simulink model "L_vs_pos_host"  (R2021b)
settings: Solver=ode1  StartTime=0.0  StopTime=inf  FixedStep=1e-3  RelTol=1e-3
InitFcn:
  | X_to_L = 1/(20*2*pi);
libraries: slrealtimeutilitieslib x1, slrealtimeiplib x1, simulink x1
settings Model: Creator=tcraddoc  LastModifiedBy=wasynczu
settings SolverCC: AlgebraicLoopSolver=TrustRegion
settings DataIOCC: ReturnWorkspaceOutputs=off
settings DebuggingCC: SFMachineParentedDataDiag=warning  ArithmeticOperatorsInVariantConditions=warning
settings SFSimCC: SimUseLocalCustomCode=off  CustomCodeUndefinedFunction=UseInterfaceOnly
settings RTWCC: RTWUseLocalCustomCode=off
settings CodeAppCC: StateflowObjectComments=on

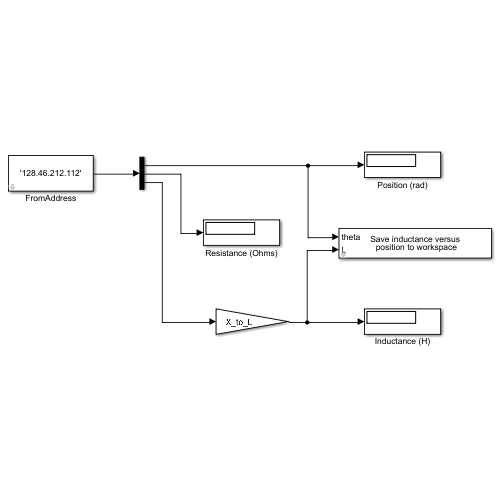
[thumbnail: Simulink's stored preview of the top-level diagram]
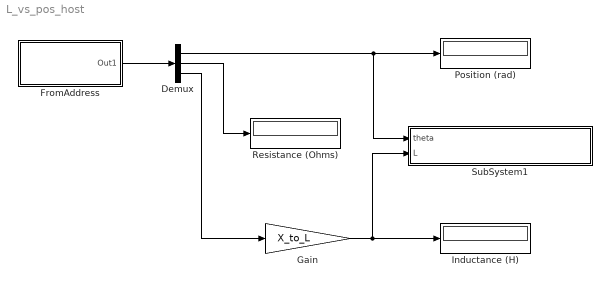
== system L_vs_pos_host ==
  Demux : Demux  Outputs=3
  FromAddress : Subsystem  mask{fromIPAddress='128.46.212.112'}
      mask prompts: fromIPAddress "From IP Address"
      mask Display: disp((get_param(gcb,'fromIPAddress')))
  Gain : Gain  Gain=X_to_L
  Inductance (H) : Display
  Position (rad) : Display
  Resistance (Ohms) : Display
  SubSystem1 : Subsystem  mask{N=10}
      mask prompts: N "Number of encoder bits"
      mask help: This block save inductance and position to the Matlab Workspace. The Matlab variables are called "position" and "inductance". The number of encoder bits should be set to that of the encoder you are using (10 in this lab)
      mask init:
      | clear inductance
      | clear position
      | dtheta = 2*pi/(2^N)
      mask Display:
      | disp('Save inductance versus\n position to workspace')
      | port_label('input', 1, 'theta')
      | port_label('input', 2, 'L')
  wires:
  FromAddress/1(Out1) -> Demux/1
  Demux/1 -> Position (rad)/1, SubSystem1/1(theta)
  Demux/3 -> Gain/1
  Gain/1 -> Inductance (H)/1, SubSystem1/2(L)
  Demux/2 -> Resistance (Ohms)/1

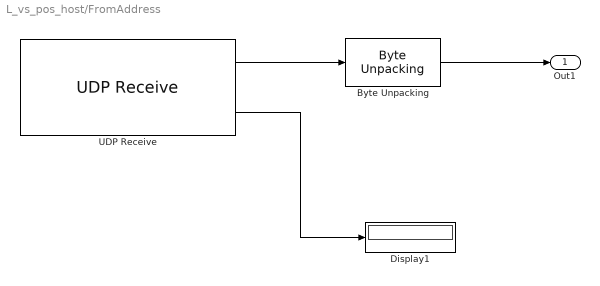
== system L_vs_pos_host/FromAddress ==
  Byte Unpacking : slrealtimeutilitieslib/Byte Unpacking  MaskUnpackedDataTypes={['double']}  MaskUnpackedDataSizes={[3]}  MaskAlignment=1
      settings: SourceProductBaseCode=XP
  Display1 : Display
  UDP Receive : slrealtimeiplib/UDP Receive  useHostTargetConn=on  ipAddress=128.46.212.188  localPort=34  rcvWidth=24  rcvFmAny=off  fmAddress=fromIPAddress  sampleTime=1e-3
      settings: SourceProductBaseCode=XP
  Out1 : Outport
  wires:
  Byte Unpacking/1 -> Out1/1
  UDP Receive/2 -> Display1/1
  UDP Receive/1 -> Byte Unpacking/1

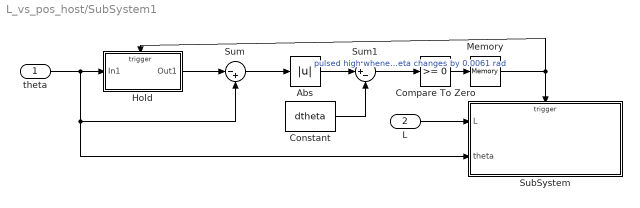
== system L_vs_pos_host/SubSystem1 ==
  theta : Inport
  L : Inport  Port=2
  Abs : Abs
  Compare To Zero : simulink/Logic and Bit Operations/Compare To Zero  relop=>=  OutDataTypeStr=boolean
  Constant : Constant  Value=dtheta
  Hold : Subsystem  TreatAsAtomicUnit=on
  Memory : Memory
  SubSystem : Subsystem  TreatAsAtomicUnit=on
  Sum : Sum  Inputs=|-+  InputSameDT=on  SaturateOnIntegerOverflow=on  OutDataTypeStr=Inherit: Same as first input
  Sum1 : Sum  Inputs=|+-  InputSameDT=on  SaturateOnIntegerOverflow=on  OutDataTypeStr=Inherit: Same as first input
  wires:
  L/1 -> SubSystem/1(L)
  theta/1 -> Hold/1(In1), Sum/2, SubSystem/2(theta)
  Hold/1(Out1) -> Sum/1
  Sum/1 -> Abs/1
  Sum1/1 -> Compare To Zero/1  "pulsed high whenever theta changes by 0.0061 rad"
  Constant/1 -> Sum1/2
  Compare To Zero/1 -> Memory/1
  Memory/1 -> SubSystem/Trigger, Hold/Trigger
  Abs/1 -> Sum1/1

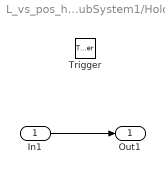
== system L_vs_pos_host/SubSystem1/Hold ==
  In1 : Inport
  Trigger : TriggerPort  VariantControl=Variant
  Out1 : Outport
  wires:
  In1/1 -> Out1/1

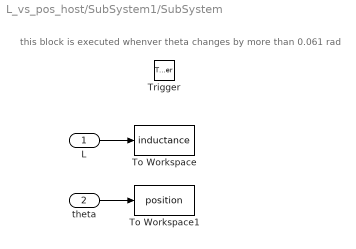
== system L_vs_pos_host/SubSystem1/SubSystem ==
  note: this block is executed whenver theta changes by more than 0.061 rad
  L : Inport
  theta : Inport  Port=2
  Trigger : TriggerPort  VariantControl=Variant
  To Workspace : ToWorkspace  VariableName=inductance  SampleTime=-1
      settings: MaxDataPoints=2^N
  To Workspace1 : ToWorkspace  VariableName=position  SampleTime=-1
      settings: MaxDataPoints=2^N
  wires:
  L/1 -> To Workspace/1
  theta/1 -> To Workspace1/1
